simulink model "sysv8"  (R2020a)
settings: Solver=VariableStepAuto  StartTime=0.0  StopTime=0.0009  RelTol=1e-3
libraries: powerlib x10, simulink_extras x3, dspswit3 x1, commsynccomp2 x1
settings Model: SimulationMode=accelerator  Creator=shang  LastModifiedBy=shang

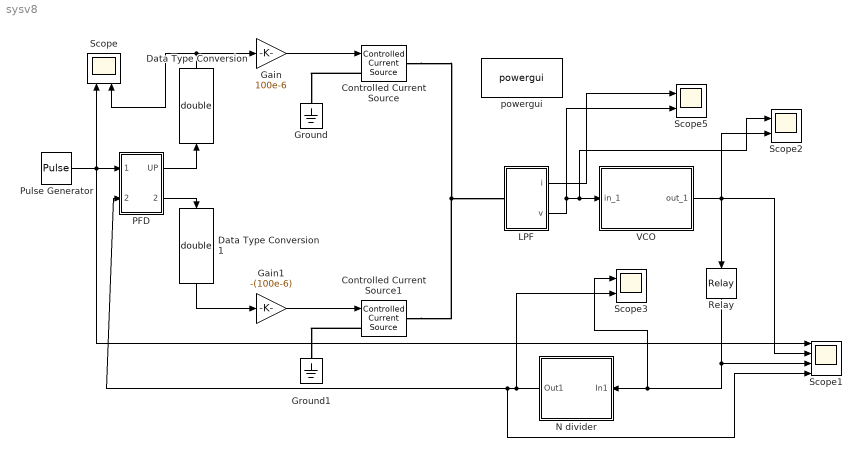
== system sysv8 ==
  Controlled Current Source : powerlib/Electrical Sources/Controlled Current Source  Initialize=on  Source_Type=DC  Amplitude=100e-6  Phase=0  Frequency=0  Measurements=Current
  Controlled Current Source1 : powerlib/Electrical Sources/Controlled Current Source  Initialize=on  Source_Type=DC  Amplitude=-(100e-6)  Phase=0  Frequency=0  Measurements=Current
  Data Type Conversion : DataTypeConversion  OutDataTypeStr=double
  Data Type Conversion1 : DataTypeConversion  OutDataTypeStr=double
  Gain : Gain  Gain=100e-6
  Gain1 : Gain  Gain=-(100e-6)
  Ground : powerlib/Elements/Ground  LConnTagsString=a
  Ground1 : powerlib/Elements/Ground  LConnTagsString=a
  LPF : Subsystem
  N divider : Subsystem
  PFD : Subsystem
  Pulse Generator : DiscretePulseGenerator  PulseType=Time based  Period=1/20*10^-6  PulseWidth=50
  Relay : Relay
  Scope{,2..3,5} (4 alike) : Scope  NumInputPorts=2
  Scope1 : Scope  NumInputPorts=4
  VCO : Subsystem
  powergui : powerlib/powergui  Priority=1  SimulationMode=Continuous  SampleTime=50e-6  frequency=60  Iterations=50  frequencyindice=0  Pbase=100e6  ErrMax=1e-4  UnitsV=kV  UnitsW=MW  buscounter=0  FunctionMessages=off  echomessages=off  EnableUseOfTLC=off  CurrentSourceSwitches=off  DisableSnubberDevices=off  DisableRonSwitches=off  DisableVfSwitches=off  DisplayEquations=off  AutomaticDiscreteSolvers=off  SolverType=Tustin/Backward Euler (TBE)  Interpol=off  ExternalGateDelay=off  methode=off  Ts=100  x0status=blocks  SPID=on  SwTol=0  HookPort=off  NonlinearTolerance=1e-4  nMaxIteration=100  ContinueOnMaxIteration=off  RestoreLinks=warning  ResistiveCurrentMeasurement=off  Frange=[0:2:500]  Ylog=off  Xlog=on  ShowGrid=off  save=off  variable=ZData  structure=logsout  ZoomFFT=off  StartTime=0.0  cycles=1  DisplayStyle=1  fundamental=60  FreqAxis=off  MaxFrequency=1000  frequencyindicesteady=1  RmsSteady=1  display=off
  wires:
  Relay/1 -> Scope3/1, N divider/1(In1), Scope1/3
  Data Type Conversion/1 -> Gain/1, Scope/2
  Data Type Conversion1/1 -> Gain1/1
  N divider/1(Out1) -> Scope3/2, Scope1/4, PFD/2(Fdiv)
  PFD/2(DN) -> Data Type Conversion1/1
  Gain1/1 -> Controlled Current Source1/1
  PFD/1(UP) -> Data Type Conversion/1
  Gain/1 -> Controlled Current Source/1
  VCO/1(out_1) -> Scope2/2, Scope1/2, Relay/1
  Pulse Generator/1 -> Scope1/1, Scope/1, PFD/1(Fref)
  LPF/2(v) -> Scope2/1, VCO/1(in_1), Scope5/2
  LPF/1(i) -> Scope5/1
  connections:
  Controlled Current Source1/RConn1 -- Controlled Current Source/RConn1 -- LPF/LConn1
  Controlled Current Source/LConn1 -- Ground/LConn1
  Controlled Current Source1/LConn1 -- Ground1/LConn1

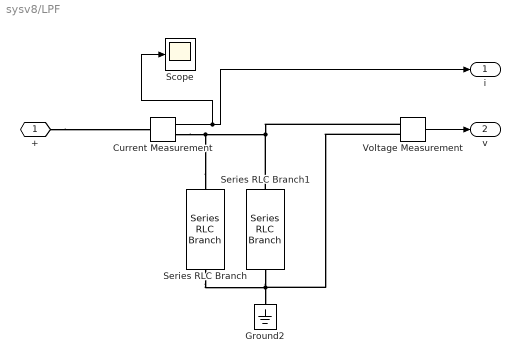
== system sysv8/LPF ==
  Current Measurement : powerlib/Measurements/Current Measurement  PhasorSimulation=off  OutputType=Complex  PSBequivalent=0
  Ground2 : powerlib/Elements/Ground  LConnTagsString=a
  Scope : Scope
  Series RLC Branch : powerlib/Elements/Series RLC Branch  LConnTagsString=__new0  RConnTagsString=__new0  BranchType=RC  Resistance=3385  Inductance=0  SetiL0=off  InitialCurrent=0  Capacitance=1.7549e-10  Setx0=off  InitialVoltage=0  Measurements=None
  Series RLC Branch1 : powerlib/Elements/Series RLC Branch  LConnTagsString=__new0  RConnTagsString=__new0  BranchType=C  Resistance=1  Inductance=1e-3  SetiL0=off  InitialCurrent=0  Capacitance=1.3574e-11  Setx0=off  InitialVoltage=0  Measurements=None
  Voltage Measurement : powerlib/Measurements/Voltage Measurement  PhasorSimulation=off  OutputType=Complex  PSBequivalent=0
  + : PMIOPort  Side=Left
  i : Outport
  v : Outport  Port=2
  wires:
  Current Measurement/1 -> Scope/1, i/1
  Voltage Measurement/1 -> v/1
  connections:
  Series RLC Branch/LConn1 -- Current Measurement/RConn1 -- Series RLC Branch1/LConn1 -- Voltage Measurement/LConn1
  Series RLC Branch1/RConn1 -- Voltage Measurement/LConn2 -- Series RLC Branch/RConn1 -- Ground2/LConn1
  +/RConn1 -- Current Measurement/LConn1

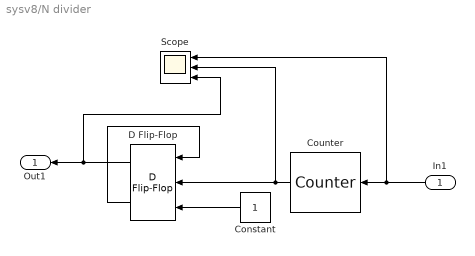
== system sysv8/N divider ==
  In1 : Inport
  Constant : Constant  OutDataTypeStr=boolean
  Counter : dspswit3/Counter  Direction=Up  CountEvent=Rising edge  CounterSize=User defined  MaxCount=24  InitialCount=0  Output=Hit  HitValue=1  ResetInput=off  SamplesPerFrame=1  Ts=1  CntDtype=double  HitDtype=Boolean
  D Flip-Flop : simulink_extras/Flip Flops/D Flip-Flop
  Scope : Scope  NumInputPorts=3
  Out1 : Outport
  wires:
  In1/1 -> Scope/1, Counter/1
  Counter/1 -> D Flip-Flop/2, Scope/2
  D Flip-Flop/1 -> Scope/3, Out1/1
  D Flip-Flop/2 -> D Flip-Flop/1
  Constant/1 -> D Flip-Flop/3

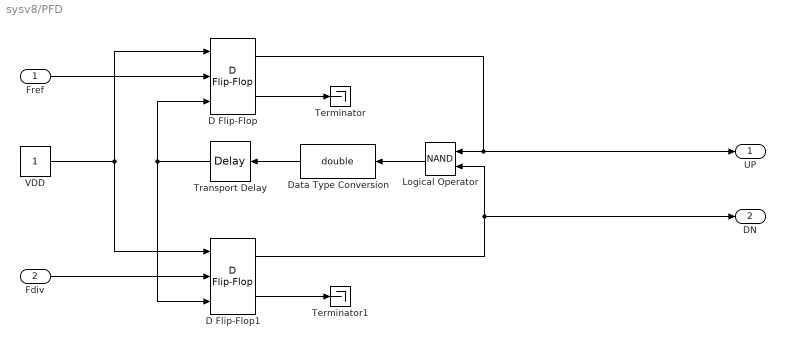
== system sysv8/PFD ==
  Fref : Inport
  Fdiv : Inport  Port=2
  D Flip-Flop : simulink_extras/Flip Flops/D Flip-Flop
  D Flip-Flop1 : simulink_extras/Flip Flops/D Flip-Flop
  Data Type Conversion : DataTypeConversion  OutDataTypeStr=double
  Logical Operator : Logic  Operator=NAND
  Terminator : Terminator
  Terminator1 : Terminator
  Transport Delay : TransportDelay  DelayTime=1*10^-11
  VDD : Constant  OutDataTypeStr=boolean
  UP : Outport  OutDataTypeStr=boolean
  DN : Outport  Port=2
  wires:
  Transport Delay/1 -> D Flip-Flop1/3, D Flip-Flop/3
  Data Type Conversion/1 -> Transport Delay/1
  D Flip-Flop1/1 -> DN/1, Logical Operator/2
  Logical Operator/1 -> Data Type Conversion/1
  VDD/1 -> D Flip-Flop1/1, D Flip-Flop/1
  D Flip-Flop1/2 -> Terminator1/1
  D Flip-Flop/2 -> Terminator/1
  Fdiv/1 -> D Flip-Flop1/2
  Fref/1 -> D Flip-Flop/2
  D Flip-Flop/1 -> UP/1, Logical Operator/1

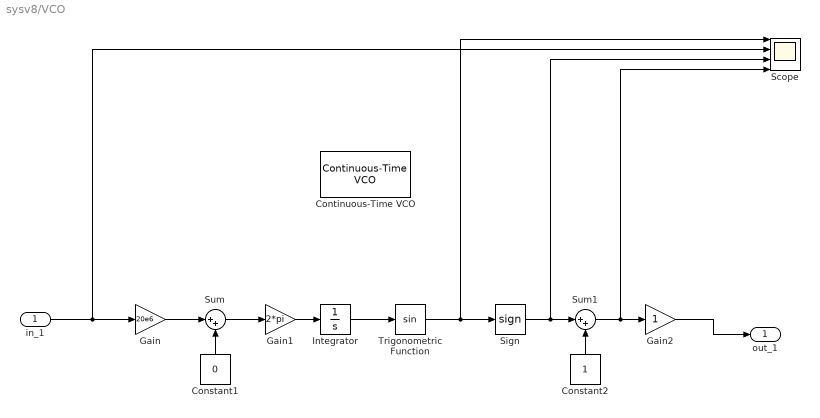
== system sysv8/VCO ==
  in_1 : Inport
  Constant1 : Constant  Value=0
  Constant2 : Constant
  Continuous-Time VCO : commsynccomp2/Continuous-Time VCO  Ac=1  Fc=0  Kc=20e6  Ph=0
      settings: SourceProductBaseCode=CM
  Gain : Gain  Gain=20e6
  Gain1 : Gain  Gain=2*pi
  Gain2 : Gain
  Integrator : Integrator  WrappedStateUpperValue=1  WrappedStateLowerValue=0
  Scope : Scope  NumInputPorts=4
  Sign : Signum
  Sum : Sum  Inputs=|++
  Sum1 : Sum  Inputs=|++
  Trigonometric Function : Trigonometry
  out_1 : Outport
  wires:
  Gain/1 -> Sum/1
  in_1/1 -> Scope/2, Gain/1
  Integrator/1 -> Trigonometric Function/1
  Constant1/1 -> Sum/2
  Trigonometric Function/1 -> Sign/1, Scope/1
  Gain1/1 -> Integrator/1
  Gain2/1 -> out_1/1
  Sum1/1 -> Scope/4, Gain2/1
  Sum/1 -> Gain1/1
  Constant2/1 -> Sum1/2
  Sign/1 -> Scope/3, Sum1/1
